simulink model "Model_openLoop"  (R2024b)
settings: Solver=ode3  StartTime=0.0  StopTime=10  FixedStep=1/30  RelTol=1e-3  EnableMultiTasking=on
undefined symbols (not defined in the file): K, valeurs_calculees
settings Model: Creator=msegui  LastModifiedBy=leofo
settings SolverCC: AlgebraicLoopSolver=TrustRegion
settings DataIOCC: LimitDataPoints=on  SaveFormat=Array  ReturnWorkspaceOutputs=off
settings OptimizationCC: ReuseModelBlockBuffer=off  LifeSpan=inf
settings DebuggingCC: UnderspecifiedInitializationDetection=Classic  MergeDetectMultiDrivingBlocksExec=none  SolverPrmCheckMsg=warning  UnconnectedInputMsg=warning  UnconnectedOutputMsg=warning  UnconnectedLineMsg=warning  SFUnexpectedBacktrackingDiag=warning  SFNoUnconditionalDefaultTransitionDiag=warning  ArithmeticOperatorsInVariantConditions=warning
settings HardwareCC: ProdBitPerPointer=32  ProdBitPerSizeT=32  ProdBitPerPtrDiffT=32  ProdLargestAtomicFloat=None  ProdIntDivRoundTo=Undefined  ProdEndianess=Unspecified  ProdWordSize=32  ProdHWDeviceType=32-bit Generic
settings ModelReferenceCC: EnableRefExpFcnMdlSchedulingChecks=on  PropagateSignalLabelsOutOfModel=off
settings SFSimCC: SimUseLocalCustomCode=off  CustomCodeUndefinedFunction=UseInterfaceOnly
settings RTWCC: RTWUseLocalCustomCode=off  GPUComputeCapability=3.5
settings CodeAppCC: StateflowObjectComments=on
settings GRTTargetCC: TargetLangStandard=C89/C90 (ANSI)
settings ConfigComp: CovMetricSettings=dw  CovSaveCumulativeToWorkspaceVar=on  CovSaveSingleToWorkspaceVar=on  CovExternalEMLEnable=off

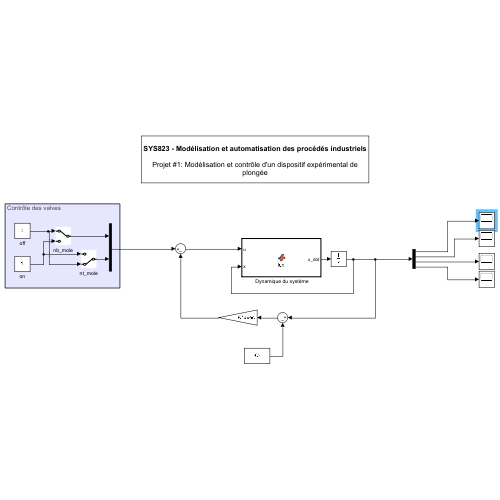
[thumbnail: Simulink's stored preview of the top-level diagram]
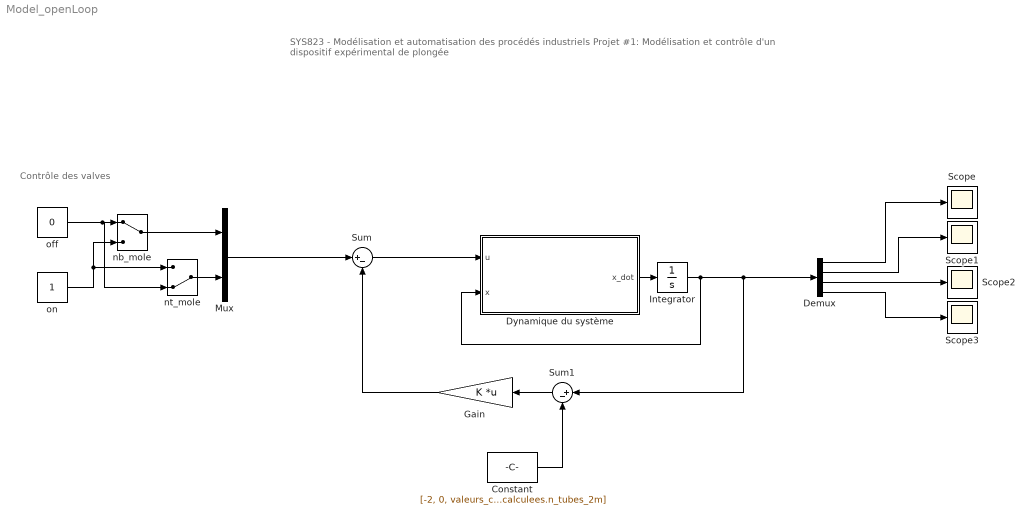
== system Model_openLoop ==
  note: SYS823 - Modélisation et automatisation des procédés industriels
      |
      | Projet #1: Modélisation et contrôle d'un dispositif expérimental de plongée
  note: Contrôle des valves
  " Dynamique du système" : MATLAB Function  TreatAsAtomicUnit=on
  Constant : Constant  Value=[-2, 0, valeurs_calculees.n_bonbonne_2m, valeurs_calculees.n_tubes_2m]
  Demux : Demux
  Gain : Gain  Gain=K  Multiplication=Matrix(K*u) (u vector)
  Integrator : Integrator  InitialCondition=[-2.2, 0, valeurs_calculees.n_bonbonne_2m, valeurs_calculees.n_tubes_2m]  UpperSaturationLimit=[inf inf inf inf]  LowerSaturationLimit=[0 -inf 0.01 0.01]
  Mux : Mux  Inputs=2
  Scope{,1..3} (4 alike) : Scope
  Sum : Sum  Inputs=|+-
  Sum1 : Sum  Inputs=|+-
  nb_mole : ManualSwitch
  nt_mole : ManualSwitch  CurrentSetting=0
  off : Constant  Value=0
  on : Constant
  wires:
  " Dynamique du système"/1(x_dot) -> Integrator/1
  nb_mole/1 -> Mux/1
  nt_mole/1 -> Mux/2
  off/1 -> nt_mole/2, nb_mole/1
  Demux/1 -> Scope/1
  on/1 -> nt_mole/1, nb_mole/2
  Sum/1 -> " Dynamique du système"/1(u)
  Mux/1 -> Sum/1
  Integrator/1 -> Sum1/1, Demux/1, " Dynamique du système"/2(x)
  Demux/2 -> Scope1/1
  Demux/3 -> Scope2/1
  Demux/4 -> Scope3/1
  Sum1/1 -> Gain/1
  Constant/1 -> Sum1/2
  Gain/1 -> Sum/2

== matlab function Model_openLoop/ Dynamique du système ==
  data: u input; x_dot output; x input
function x_dot = fcn(u, x)

%%% Initialisation du vecteur de sortie
x_dot = zeros(4,1);

%%% Récupération des états
z  = x(1);
z_p = x(2);
n_bonbonne = x(3);
n_tubes = x(4);

u_bonbonne = u(1);
u_tubes = u(2);

x_dot(1) = z_p;
x_dot(2) = (9810*((87416213640596439521297*pi)/9007199254740992000000000 - (13721256126300354489*n_tubes)/(5629499534213120*(9810*z - 101300))))/((4174345133550735*n_bonbonne)/144115188075855872 + (12523035400652205*n_tubes)/144115188075855872 + (1722577179000855092860691*pi)/180143985094819840000000 + 25/2) - 981/100;
x_dot(3) = -(u_bonbonne*((68606280631501772445*n_bonbonne)/281474976710656 + 4905*z - ((2804281720812634948689375*n_tubes)/(462344639479808*pi) + (9810*z - 2535443/25)^2)^(1/2)/2 - 2535443/50)^(1/2))/5000;
x_dot(4) = (u_bonbonne*((68606280631501772445*n_bonbonne)/281474976710656 + 4905*z - ((2804281720812634948689375*n_tubes)/(462344639479808*pi) + (9810*z - 2535443/25)^2)^(1/2)/2 - 2535443/50)^(1/2))/5000 - (u_tubes*(4905*z + ((2804281720812634948689375*n_tubes)/(462344639479808*pi) + (9810*z - 2535443/25)^2)^(1/2)/2 - 2529557/50)^(1/2))/5000;


end
